simulink model "gm_wlanhdlTimeAndFrequencySynchronization"  (R2025a)
settings: Solver=FixedStepDiscrete  StartTime=0.0  StopTime=stopTime  RelTol=1e-3
InitFcn:
  | wlanFrontEndInit;
undefined symbols (not defined in the file or in its folder): a, b, c, Hd, wlanConfig
libraries: simulink x95, hdlsllib x16, hdlmdlgenlib x12, dspsrcs4 x3, dspsigops x3, dsphdlsigops2 x2, dsphdlfiltering2 x2
(part 10 of 11)

== system gm_wlanhdlTimeAndFrequencySynchronization/WLANTimeAndFrequencySynchronization/Fine CFO Estimation and Correction/Fine CFO Estimation/Iteration8 ==
  xin : Inport  OutDataTypeStr=fixdt(1, 32, 19)  SampleTime=6.25e-09
  yin : Inport  Port=2  OutDataTypeStr=fixdt(1, 32, 19)  SampleTime=6.25e-09
  zin : Inport  Port=3  OutDataTypeStr=fixdt(1, 34, 33)  SampleTime=6.25e-09
  lut_value : Inport  Port=4  OutDataTypeStr=fixdt(0, 31, 33)  SampleTime=6.25e-09
  idx : Inport  Port=5  OutDataTypeStr=fixdt(0, 6, 0)  SampleTime=6.25e-09
  MuxX : Switch  Criteria=u2 ~= 0  Threshold="fi(0,0,1,0,\"hex\",\"0\")"  OutDataTypeStr=fixdt(1, 32, 19)  SampleTime=6.25e-09  SaturateOnIntegerOverflow=off  InputSameDT=off
  MuxY : Switch  Criteria=u2 ~= 0  Threshold="fi(0,0,1,0,\"hex\",\"0\")"  OutDataTypeStr=fixdt(1, 32, 19)  SampleTime=6.25e-09  SaturateOnIntegerOverflow=off  InputSameDT=off
  MuxZ : Switch  Criteria=u2 ~= 0  Threshold="fi(0,0,1,0,\"hex\",\"0\")"  OutDataTypeStr=fixdt(1, 34, 33)  SampleTime=6.25e-09  SaturateOnIntegerOverflow=off  InputSameDT=off
  XAdder : Sum  OutDataTypeStr=fixdt(1, 32, 19)  SampleTime=6.25e-09
  XSubtractor : Sum  Inputs=+-  OutDataTypeStr=fixdt(1, 32, 19)  AccumDataTypeStr=fixdt(1, 32, 19)  SampleTime=6.25e-09
  YAdder : Sum  OutDataTypeStr=fixdt(1, 32, 19)  SampleTime=6.25e-09
  YSub : Sum  Inputs=+-  OutDataTypeStr=fixdt(1, 32, 19)  AccumDataTypeStr=fixdt(1, 32, 19)  SampleTime=6.25e-09
  ZAdder : Sum  OutDataTypeStr=fixdt(1, 34, 33)  SampleTime=6.25e-09
  ZSub : Sum  Inputs=+-  OutDataTypeStr=fixdt(1, 34, 33)  AccumDataTypeStr=fixdt(1, 34, 33)  SampleTime=6.25e-09
  compare : simulink/Logic and Bit Operations/Compare To Constant  relop=<  const=double(0)  OutDataTypeStr=boolean
  dynamic_shift : ArithShift  BitShiftNumberSource=Input port  BitShiftDirection=Right
      settings: InputPortMap=u0,p1
  dynamic_shift1 : ArithShift  BitShiftNumberSource=Input port  BitShiftDirection=Right
      settings: InputPortMap=u0,p1
  rd_{0..9} (10 alike) : Delay  DelayLength=double(1)  InitialCondition=0  SampleTime=6.25e-09
  xout : Outport  OutDataTypeStr=fixdt(1, 32, 19)  SampleTime=6.25e-09
  yout : Outport  Port=2  OutDataTypeStr=fixdt(1, 32, 19)  SampleTime=6.25e-09
  zout : Outport  Port=3  OutDataTypeStr=fixdt(1, 34, 33)  SampleTime=6.25e-09
  wires:
  rd_3/1 -> MuxZ/2, MuxY/2, MuxX/2
  rd_2/1 -> MuxX/1
  rd_6/1 -> MuxY/3
  ZAdder/1 -> rd_9/1
  ZSub/1 -> rd_8/1
  yin/1 -> rd_1/1
  MuxZ/1 -> zout/1
  MuxX/1 -> xout/1
  XAdder/1 -> rd_4/1
  idx/1 -> dynamic_shift/2, dynamic_shift1/2
  xin/1 -> rd_0/1
  rd_9/1 -> MuxZ/3
  zin/1 -> rd_7/1
  rd_1/1 -> compare/1, dynamic_shift1/1, YSub/1, YAdder/1
  rd_4/1 -> MuxX/3
  YSub/1 -> rd_6/1
  rd_0/1 -> dynamic_shift/1, XSubtractor/1, XAdder/1
  dynamic_shift/1 -> YAdder/2, YSub/2
  XSubtractor/1 -> rd_2/1
  compare/1 -> rd_3/1
  rd_8/1 -> MuxZ/1
  YAdder/1 -> rd_5/1
  rd_7/1 -> ZSub/1, ZAdder/1
  MuxY/1 -> yout/1
  rd_5/1 -> MuxY/1
  dynamic_shift1/1 -> XSubtractor/2, XAdder/2
  lut_value/1 -> ZSub/2, ZAdder/2

== system gm_wlanhdlTimeAndFrequencySynchronization/WLANTimeAndFrequencySynchronization/Fine CFO Estimation and Correction/Fine CFO Estimation/Iteration9 ==
  xin : Inport  OutDataTypeStr=fixdt(1, 32, 19)  SampleTime=6.25e-09
  yin : Inport  Port=2  OutDataTypeStr=fixdt(1, 32, 19)  SampleTime=6.25e-09
  zin : Inport  Port=3  OutDataTypeStr=fixdt(1, 34, 33)  SampleTime=6.25e-09
  lut_value : Inport  Port=4  OutDataTypeStr=fixdt(0, 31, 33)  SampleTime=6.25e-09
  idx : Inport  Port=5  OutDataTypeStr=fixdt(0, 6, 0)  SampleTime=6.25e-09
  MuxX : Switch  Criteria=u2 ~= 0  Threshold="fi(0,0,1,0,\"hex\",\"0\")"  OutDataTypeStr=fixdt(1, 32, 19)  SampleTime=6.25e-09  SaturateOnIntegerOverflow=off  InputSameDT=off
  MuxY : Switch  Criteria=u2 ~= 0  Threshold="fi(0,0,1,0,\"hex\",\"0\")"  OutDataTypeStr=fixdt(1, 32, 19)  SampleTime=6.25e-09  SaturateOnIntegerOverflow=off  InputSameDT=off
  MuxZ : Switch  Criteria=u2 ~= 0  Threshold="fi(0,0,1,0,\"hex\",\"0\")"  OutDataTypeStr=fixdt(1, 34, 33)  SampleTime=6.25e-09  SaturateOnIntegerOverflow=off  InputSameDT=off
  XAdder : Sum  OutDataTypeStr=fixdt(1, 32, 19)  SampleTime=6.25e-09
  XSubtractor : Sum  Inputs=+-  OutDataTypeStr=fixdt(1, 32, 19)  AccumDataTypeStr=fixdt(1, 32, 19)  SampleTime=6.25e-09
  YAdder : Sum  OutDataTypeStr=fixdt(1, 32, 19)  SampleTime=6.25e-09
  YSub : Sum  Inputs=+-  OutDataTypeStr=fixdt(1, 32, 19)  AccumDataTypeStr=fixdt(1, 32, 19)  SampleTime=6.25e-09
  ZAdder : Sum  OutDataTypeStr=fixdt(1, 34, 33)  SampleTime=6.25e-09
  ZSub : Sum  Inputs=+-  OutDataTypeStr=fixdt(1, 34, 33)  AccumDataTypeStr=fixdt(1, 34, 33)  SampleTime=6.25e-09
  compare : simulink/Logic and Bit Operations/Compare To Constant  relop=<  const=double(0)  OutDataTypeStr=boolean
  dynamic_shift : ArithShift  BitShiftNumberSource=Input port  BitShiftDirection=Right
      settings: InputPortMap=u0,p1
  dynamic_shift1 : ArithShift  BitShiftNumberSource=Input port  BitShiftDirection=Right
      settings: InputPortMap=u0,p1
  rd_{0..9} (10 alike) : Delay  DelayLength=double(1)  InitialCondition=0  SampleTime=6.25e-09
  xout : Outport  OutDataTypeStr=fixdt(1, 32, 19)  SampleTime=6.25e-09
  yout : Outport  Port=2  OutDataTypeStr=fixdt(1, 32, 19)  SampleTime=6.25e-09
  zout : Outport  Port=3  OutDataTypeStr=fixdt(1, 34, 33)  SampleTime=6.25e-09
  wires:
  MuxX/1 -> xout/1
  MuxZ/1 -> zout/1
  rd_4/1 -> MuxX/3
  rd_3/1 -> MuxZ/2, MuxX/2, MuxY/2
  rd_5/1 -> MuxY/1
  rd_8/1 -> MuxZ/1
  MuxY/1 -> yout/1
  XAdder/1 -> rd_4/1
  rd_9/1 -> MuxZ/3
  XSubtractor/1 -> rd_2/1
  yin/1 -> rd_1/1
  zin/1 -> rd_7/1
  YAdder/1 -> rd_5/1
  rd_1/1 -> compare/1, dynamic_shift1/1, YAdder/1, YSub/1
  rd_6/1 -> MuxY/3
  idx/1 -> dynamic_shift1/2, dynamic_shift/2
  rd_2/1 -> MuxX/1
  rd_7/1 -> ZSub/1, ZAdder/1
  lut_value/1 -> ZAdder/2, ZSub/2
  dynamic_shift1/1 -> XAdder/2, XSubtractor/2
  YSub/1 -> rd_6/1
  xin/1 -> rd_0/1
  rd_0/1 -> dynamic_shift/1, XSubtractor/1, XAdder/1
  compare/1 -> rd_3/1
  dynamic_shift/1 -> YSub/2, YAdder/2
  ZSub/1 -> rd_8/1
  ZAdder/1 -> rd_9/1

== system gm_wlanhdlTimeAndFrequencySynchronization/WLANTimeAndFrequencySynchronization/Fine CFO Estimation and Correction/Fine CFO Estimation/QuadrantCorrection ==
  zin : Inport  OutDataTypeStr=fixdt(1, 34, 33)  SampleTime=6.25e-09
  QA_Control : Inport  Port=2  OutDataTypeStr=fixdt(0, 5, 0)  SampleTime=6.25e-09
  Negation : Gain  Gain="fi(0,1,2,0,\"hex\",\"3\")"  ParamDataTypeStr=fixdt(1, 2, 0)  OutDataTypeStr=fixdt(1, 34, 33)  SampleTime=6.25e-09
  adder : Sum  OutDataTypeStr=fixdt(1, 34, 33)  SampleTime=6.25e-09
  dtc : hdlmdlgenlib/Buffer
  extract : simulink/Logic and Bit Operations/Extract Bits  bitsToExtract=Range of bits  numBits=8  bitIdxRange=[2 2]  outScalingMode=Treat bit field as an integer
  extract1 : simulink/Logic and Bit Operations/Extract Bits  bitsToExtract=Range of bits  numBits=8  bitIdxRange=[0 1]  outScalingMode=Treat bit field as an integer
  mux : MultiPortSwitch  DataPortOrder=Zero-based contiguous  Inputs=2  DiagnosticForDefault=None  zeroidx=on  OutDataTypeStr=fixdt(1, 34, 33)  SampleTime=6.25e-09  SaturateOnIntegerOverflow=off  InputSameDT=off
  mux1 : MultiPortSwitch  DataPortOrder=Zero-based contiguous  Inputs=4  DiagnosticForDefault=None  zeroidx=on  OutDataTypeStr=fixdt(1, 34, 33)  SampleTime=6.25e-09  SaturateOnIntegerOverflow=off  InputSameDT=off
  mux2 : MultiPortSwitch  DataPortOrder=Zero-based contiguous  Inputs=2  DiagnosticForDefault=None  zeroidx=on  OutDataTypeStr=fixdt(1, 34, 33)  SampleTime=6.25e-09  SaturateOnIntegerOverflow=off  InputSameDT=off
  mux3 : MultiPortSwitch  DataPortOrder=Zero-based contiguous  Inputs=2  DiagnosticForDefault=None  zeroidx=on  OutDataTypeStr=fixdt(1, 34, 33)  SampleTime=6.25e-09  SaturateOnIntegerOverflow=off  InputSameDT=off
  mux6out_wire : hdlmdlgenlib/Buffer
  pidivtwoconstant : Constant  Value=0.5  OutDataTypeStr=fixdt(1, 34, 33)  SampleTime=6.25e-09
  pidivtwoconstant1 : Constant  Value=0.999999999883584678173065185546875  OutDataTypeStr=fixdt(1, 34, 33)  SampleTime=6.25e-09
  pidivtwoconstant2 : Constant  Value=-1  OutDataTypeStr=fixdt(1, 34, 33)  SampleTime=6.25e-09
  pidivtwoconstant3 : Constant  Value=0  OutDataTypeStr=fixdt(1, 34, 33)  SampleTime=6.25e-09
  pidivtwosub : Sum  Inputs=+-  OutDataTypeStr=fixdt(1, 34, 33)  AccumDataTypeStr=fixdt(1, 34, 33)  SampleTime=6.25e-09
  rd_{0,2..3,6..7} (5 alike) : Delay  DelayLength=double(1)  InitialCondition=0  SampleTime=6.25e-09
  rd_{1,4..5,8..9} (5 alike) : Delay  DelayLength=double(2)  InitialCondition=0  SampleTime=6.25e-09
  slice : hdlsllib/Logic and Bit Operations/Bit Slice  lidx=double(3)  ridx=double(3)
  slice1 : hdlsllib/Logic and Bit Operations/Bit Slice  lidx=double(4)  ridx=double(4)
  subfmux : Sum  Inputs=+-  OutDataTypeStr=fixdt(1, 34, 33)  AccumDataTypeStr=fixdt(1, 34, 33)  SampleTime=6.25e-09
  zout : Outport  OutDataTypeStr=fixdt(1, 34, 33)  SampleTime=6.25e-09
  wires:
  mux6out_wire/1 -> zout/1
  pidivtwoconstant2/1 -> adder/1
  Negation/1 -> rd_7/1
  extract1/1 -> rd_5/1
  pidivtwosub/1 -> mux/2
  rd_2/1 -> dtc/1
  extract/1 -> mux/1
  slice1/1 -> rd_1/1
  rd_7/1 -> mux1/3
  mux/1 -> rd_3/1, adder/2, subfmux/2
  rd_5/1 -> mux1/1
  rd_9/1 -> mux1/5
  mux1/1 -> mux2/2
  dtc/1 -> pidivtwosub/2, mux/3
  slice/1 -> rd_4/1
  pidivtwoconstant/1 -> pidivtwosub/1
  mux3/1 -> mux6out_wire/1
  rd_0/1 -> extract/1, slice/1, slice1/1, extract1/1
  rd_6/1 -> mux1/2
  QA_Control/1 -> rd_0/1
  rd_3/1 -> rd_6/1, Negation/1
  pidivtwoconstant1/1 -> subfmux/1, mux2/3
  adder/1 -> rd_9/1
  pidivtwoconstant3/1 -> mux3/3
  subfmux/1 -> rd_8/1
  rd_8/1 -> mux1/4
  zin/1 -> rd_2/1
  rd_1/1 -> mux3/1
  rd_4/1 -> mux2/1
  mux2/1 -> mux3/2

== system gm_wlanhdlTimeAndFrequencySynchronization/WLANTimeAndFrequencySynchronization/Fine CFO Estimation and Correction/Fine CFO Estimation/QuadrantMapper ==
  xin : Inport  OutDataTypeStr=fixdt(1, 32, 19)  SampleTime=5e-08
  yin : Inport  Port=2  OutDataTypeStr=fixdt(1, 32, 19)  SampleTime=5e-08
  Delayin1 : UnitDelay  InitialCondition=double(0)  SampleTime=5e-08
  Delayin11 : RateTransition  InitialCondition=double(0)  OutPortSampleTimeOpt=Multiple of input port sample time  OutPortSampleTimeMultiple=8
  Delayin2 : UnitDelay  InitialCondition=double(0)  SampleTime=5e-08
  Delayin21 : RateTransition  InitialCondition=double(0)  OutPortSampleTimeOpt=Multiple of input port sample time  OutPortSampleTimeMultiple=8
  DelayxAbs : RateTransition  InitialCondition=double(0)  OutPortSampleTimeOpt=Multiple of input port sample time  OutPortSampleTimeMultiple=8
  DelayxAbs_absorbed : Delay  DelayLength=0
  DelayyAbs : RateTransition  InitialCondition=double(0)  OutPortSampleTimeOpt=Multiple of input port sample time  OutPortSampleTimeMultiple=8
  DelayyAbs_absorbed : Delay  DelayLength=0
  abs : Abs  SampleTime=6.25e-09  OutDataTypeStr=fixdt(1, 32, 19)  SaturateOnIntegerOverflow=off
  abs1 : Abs  SampleTime=6.25e-09  OutDataTypeStr=fixdt(1, 32, 19)  SaturateOnIntegerOverflow=off
  and : Logic  AllPortsSameDT=off  OutDataTypeStr=fixdt(0, 1, 0)  SampleTime=6.25e-09
  and1 : Logic  AllPortsSameDT=off  OutDataTypeStr=fixdt(0, 1, 0)  SampleTime=6.25e-09
  compare : simulink/Logic and Bit Operations/Compare To Constant  relop=<  const=double(0)  OutDataTypeStr=boolean
  compare1 : simulink/Logic and Bit Operations/Compare To Constant  relop===  const=double(0)  OutDataTypeStr=boolean
  compare2 : simulink/Logic and Bit Operations/Compare To Constant  relop=>=  const=double(0)  OutDataTypeStr=boolean
  compare3 : simulink/Logic and Bit Operations/Compare To Constant  relop=<  const=double(0)  OutDataTypeStr=boolean
  concatQCControl : hdlsllib/Logic and Bit Operations/Bit Concat  numInputs=5
  crp_out_delay : Delay  DelayLength=double(1)  InitialCondition=0  SampleTime=6.25e-09
  crp_out_delay1 : Delay  DelayLength=double(1)  InitialCondition=0  SampleTime=6.25e-09
  dtc : hdlmdlgenlib/Buffer
  dtc1 : hdlmdlgenlib/Buffer
  in0_repeat : RateTransition  Integrity=off  Deterministic=off  OutPortSampleTimeOpt=Multiple of input port sample time  OutPortSampleTimeMultiple=1/8
  in0_repeat1 : RateTransition  Integrity=off  Deterministic=off  OutPortSampleTimeOpt=Multiple of input port sample time  OutPortSampleTimeMultiple=1/8
  in1_repeat : RateTransition  Integrity=off  Deterministic=off  OutPortSampleTimeOpt=Multiple of input port sample time  OutPortSampleTimeMultiple=1/8
  in1_repeat1 : RateTransition  Integrity=off  Deterministic=off  OutPortSampleTimeOpt=Multiple of input port sample time  OutPortSampleTimeMultiple=1/8
  in2_repeat : RateTransition  Integrity=off  Deterministic=off  OutPortSampleTimeOpt=Multiple of input port sample time  OutPortSampleTimeMultiple=1/8
  in3_repeat : RateTransition  Integrity=off  Deterministic=off  OutPortSampleTimeOpt=Multiple of input port sample time  OutPortSampleTimeMultiple=1/8
  mux : MultiPortSwitch  DataPortOrder=Zero-based contiguous  Inputs=2  DiagnosticForDefault=None  zeroidx=on  OutDataTypeStr=fixdt(1, 32, 19)  SampleTime=6.25e-09  SaturateOnIntegerOverflow=off  InputSameDT=off
  mux1 : MultiPortSwitch  DataPortOrder=Zero-based contiguous  Inputs=2  DiagnosticForDefault=None  zeroidx=on  OutDataTypeStr=fixdt(1, 32, 19)  SampleTime=6.25e-09  SaturateOnIntegerOverflow=off  InputSameDT=off
  qcControl_wire : hdlmdlgenlib/Buffer
  rd_{0..10,41} (12 alike) : Delay  DelayLength=double(1)  InitialCondition=0  SampleTime=6.25e-09
  rd_01 : Delay  DelayLength=double(1)  InitialCondition=0  SampleTime=6.25e-09
  relop : RelationalOperator  Operator=>  OutDataTypeStr=fixdt(0, 1, 0)  SampleTime=6.25e-09
  xout : Outport  OutDataTypeStr=fixdt(1, 32, 19)  SampleTime=6.25e-09
  yout : Outport  Port=2  OutDataTypeStr=fixdt(1, 32, 19)  SampleTime=6.25e-09
  QA_Control : Outport  Port=3  OutDataTypeStr=fixdt(0, 5, 0)  SampleTime=6.25e-09
  wires:
  rd_9/1 -> mux/2, mux1/3
  rd_7/1 -> concatQCControl/3, mux/1, mux1/1
  and/1 -> concatQCControl/2
  mux/1 -> dtc/1
  and1/1 -> concatQCControl/1
  relop/1 -> rd_7/1
  rd_10/1 -> mux/3, mux1/2
  rd_6/1 -> relop/2, rd_10/1
  rd_4/1 -> and/2, concatQCControl/4
  crp_out_delay/1 -> DelayyAbs/1
  abs/1 -> crp_out_delay/1
  concatQCControl/1 -> qcControl_wire/1
  abs1/1 -> crp_out_delay1/1
  yin/1 -> in0_repeat1/1
  rd_3/1 -> and1/2
  DelayxAbs/1 -> DelayxAbs_absorbed/1
  Delayin11/1 -> Delayin1/1
  rd_41/1 -> abs1/1
  compare1/1 -> rd_1/1
  DelayyAbs/1 -> DelayyAbs_absorbed/1
  dtc/1 -> yout/1
  crp_out_delay1/1 -> DelayxAbs/1
  in0_repeat1/1 -> Delayin21/1, rd_01/1
  in1_repeat1/1 -> rd_41/1, Delayin11/1
  rd_01/1 -> abs/1
  dtc1/1 -> xout/1
  rd_8/1 -> concatQCControl/5
  rd_1/1 -> and/1, and1/1
  Delayin2/1 -> in1_repeat/1
  xin/1 -> in1_repeat1/1
  in3_repeat/1 -> rd_6/1
  Delayin1/1 -> in0_repeat/1
  in0_repeat/1 -> rd_2/1
  qcControl_wire/1 -> QA_Control/1
  in1_repeat/1 -> rd_0/1
  compare2/1 -> rd_3/1
  DelayxAbs_absorbed/1 -> in2_repeat/1
  DelayyAbs_absorbed/1 -> in3_repeat/1
  rd_2/1 -> compare/1, compare2/1
  rd_0/1 -> compare1/1, compare3/1
  in2_repeat/1 -> rd_5/1
  compare/1 -> rd_4/1
  mux1/1 -> dtc1/1
  compare3/1 -> rd_8/1
  Delayin21/1 -> Delayin2/1
  rd_5/1 -> relop/1, rd_9/1

== system gm_wlanhdlTimeAndFrequencySynchronization/WLANTimeAndFrequencySynchronization/Fine CFO Estimation and Correction/Fine CFO Estimation/sample FreqOff ==
  freqOffIn : Inport  OutDataTypeStr=fixdt(1, 34, 33)  PortDimensions=1  SampleTime=5e-08
  enb : Inport  Port=2  OutDataTypeStr=boolean  PortDimensions=1  SampleTime=5e-08
  rst : Inport  Port=3  OutDataTypeStr=boolean  PortDimensions=1  SampleTime=5e-08
  Sample FreqOff : MATLAB Function  TreatAsAtomicUnit=on
  freqOffOut : Outport  SampleTime=5e-08  VectorParamsAs1DForOutWhenUnconnected=off
  wires:
  freqOffIn/1 -> Sample FreqOff/1(freqOffIn)
  enb/1 -> Sample FreqOff/2(enb)
  rst/1 -> Sample FreqOff/3(rst)
  Sample FreqOff/1(freqOffOut) -> freqOffOut/1

== system gm_wlanhdlTimeAndFrequencySynchronization/WLANTimeAndFrequencySynchronization/Fine Time Sync/Correlator/MagnitudeSquared ==
  dataIn : Inport  OutDataTypeStr=fixdt(1, 37, 26)  PortDimensions=1  SampleTime=5e-08
      settings: SignalType=complex
  validIn : Inport  Port=2  OutDataTypeStr=boolean  PortDimensions=1  SampleTime=5e-08
  Add : Sum  OutDataTypeStr=fixdt(1, 33, 16)  AccumDataTypeStr=fixdt(1, 33, 16)  SampleTime=6.25e-09
  Complex to Real-Imag : ComplexToRealImag  SampleTime=5e-08
  Data Type  Conversion : DataTypeConversion  OutDataTypeStr=fixdt(1, 16, 8)  SampleTime=5e-08  SaturateOnIntegerOverflow=off  RndMeth=Floor
  Data Type  Conversion1 : DataTypeConversion  OutDataTypeStr=fixdt(1, 32, 15)  SampleTime=6.25e-09  SaturateOnIntegerOverflow=off  RndMeth=Floor
  Delay1 : Delay  DelayLength=double(2)  InitialCondition=0  SampleTime=5e-08
  Delay3 : Delay  DelayLength=double(2)  InitialCondition=0  SampleTime=5e-08
  Delay4 : RateTransition  InitialCondition=double(0)  OutPortSampleTimeOpt=Multiple of input port sample time  OutPortSampleTimeMultiple=8
  Delay4_absorbed : Delay  DelayLength=0
  Delay5 : RateTransition  InitialCondition=double(0)  OutPortSampleTimeOpt=Multiple of input port sample time  OutPortSampleTimeMultiple=8
  Delay5_absorbed : Delay  DelayLength=0
  Delay6 : Delay  DelayLength=double(3)  InitialCondition=0  SampleTime=5e-08
  Delay61 : RateTransition  InitialCondition=double(0)  OutPortSampleTimeOpt=Multiple of input port sample time  OutPortSampleTimeMultiple=8
  HwModeRegister{,1..3} (4 alike) : Delay  DelayLength=double(1)  InitialCondition=0  SampleTime=6.25e-09
  PipelineRegister : Delay  DelayLength=double(1)  InitialCondition=0  SampleTime=6.25e-09
  PipelineRegister1 : Delay  DelayLength=double(1)  InitialCondition=0  SampleTime=6.25e-09
  Product1 : Product  Inputs=**  OutDataTypeStr=fixdt(1, 32, 16)  SampleTime=6.25e-09
  Product4 : Product  Inputs=**  OutDataTypeStr=fixdt(1, 32, 16)  SampleTime=6.25e-09
  crp_out_delay : Delay  DelayLength=double(1)  InitialCondition=0  SampleTime=6.25e-09
  crp_out_delay1 : Delay  DelayLength=double(1)  InitialCondition=0  SampleTime=6.25e-09
  in0_repeat : RateTransition  Integrity=off  Deterministic=off  OutPortSampleTimeOpt=Multiple of input port sample time  OutPortSampleTimeMultiple=1/8
  in0_repeat1 : RateTransition  Integrity=off  Deterministic=off  OutPortSampleTimeOpt=Multiple of input port sample time  OutPortSampleTimeMultiple=1/8
  in1_repeat : RateTransition  Integrity=off  Deterministic=off  OutPortSampleTimeOpt=Multiple of input port sample time  OutPortSampleTimeMultiple=1/8
  in1_repeat1 : RateTransition  Integrity=off  Deterministic=off  OutPortSampleTimeOpt=Multiple of input port sample time  OutPortSampleTimeMultiple=1/8
  in2_repeat : RateTransition  Integrity=off  Deterministic=off  OutPortSampleTimeOpt=Multiple of input port sample time  OutPortSampleTimeMultiple=1/8
  in2_repeat1 : RateTransition  Integrity=off  Deterministic=off  OutPortSampleTimeOpt=Multiple of input port sample time  OutPortSampleTimeMultiple=1/8
  in3_repeat : RateTransition  Integrity=off  Deterministic=off  OutPortSampleTimeOpt=Multiple of input port sample time  OutPortSampleTimeMultiple=1/8
  rd_{0..4,11} (6 alike) : Delay  DelayLength=double(1)  InitialCondition=0  SampleTime=6.25e-09
  dataOut : Outport  SampleTime=6.25e-09  VectorParamsAs1DForOutWhenUnconnected=off
  validOut : Outport  Port=2  SampleTime=5e-08  VectorParamsAs1DForOutWhenUnconnected=off
  wires:
  in2_repeat/1 -> rd_2/1
  in1_repeat/1 -> rd_1/1
  Delay5_absorbed/1 -> in2_repeat/1
  in2_repeat1/1 -> rd_3/1
  rd_11/1 -> HwModeRegister1/1
  Delay6/1 -> validOut/1
  Data Type  Conversion1/1 -> dataOut/1
  Delay3/1 -> in2_repeat1/1, in3_repeat/1
  in0_repeat/1 -> Delay61/1
  HwModeRegister1/1 -> Product4/2
  in0_repeat1/1 -> rd_0/1
  crp_out_delay/1 -> Delay4/1
  Delay4_absorbed/1 -> in1_repeat/1
  Delay5/1 -> Delay5_absorbed/1
  in3_repeat/1 -> rd_4/1
  Delay1/1 -> in0_repeat1/1, in1_repeat1/1
  Complex to Real-Imag/2 -> Delay3/1
  Complex to Real-Imag/1 -> Delay1/1
  Add/1 -> Data Type  Conversion1/1
  dataIn/1 -> Data Type  Conversion/1
  Data Type  Conversion/1 -> Complex to Real-Imag/1
  rd_2/1 -> Add/2
  validIn/1 -> in0_repeat/1
  HwModeRegister3/1 -> Product1/2
  HwModeRegister/1 -> Product4/1
  crp_out_delay1/1 -> Delay5/1
  in1_repeat1/1 -> rd_11/1
  Delay61/1 -> Delay6/1
  Product1/1 -> PipelineRegister1/1
  PipelineRegister1/1 -> crp_out_delay1/1
  rd_0/1 -> HwModeRegister/1
  rd_1/1 -> Add/1
  rd_3/1 -> HwModeRegister2/1
  rd_4/1 -> HwModeRegister3/1
  Delay4/1 -> Delay4_absorbed/1
  HwModeRegister2/1 -> Product1/1
  PipelineRegister/1 -> crp_out_delay/1
  Product4/1 -> PipelineRegister/1

== system gm_wlanhdlTimeAndFrequencySynchronization/WLANTimeAndFrequencySynchronization/Fine Time Sync/Correlator/corrFilter ==
  dataIn : Inport  OutDataTypeStr=fixdt(1, 16, 12)  PortDimensions=1  SampleTime=5e-08
      settings: SignalType=complex
  validIn : Inport  Port=2  OutDataTypeStr=boolean  PortDimensions=1  SampleTime=5e-08
  rst : Inport  Port=3  OutDataTypeStr=boolean  PortDimensions=1  SampleTime=5e-08
  C1 : dsphdlfiltering2/Discrete FIR Filter  NumeratorSource=Property  Numerator=conj(flipud(wlanConfig.lltf(1:wlanConfig.corrLen))).'  NumeratorPrototype=[ 0.5, 0.5 ]  FilterStructure=Partly serial systolic  SerializationOption=Minimum number of cycles between valid input samples  NumCycles=filterUpsampleFactor  NumberOfMultipliers=2  SimulateUsing=Code generation  roundingMode=Floor  overflowMode=off  CoefficientsDataTypeStr=fixdt(1,16,14)  ResetInputPort=on  HDLGlobalReset=off  CoeffMultiplier=Multiplier  UseMultForPow2Coeff=on  FrameInputSymmOptim=off
  C1_term2 : Terminator
  Delay : Delay  DelayLength=double(7)  InitialCondition=0  SampleTime=6.25e-09
  Delay1 : Delay  DelayLength=double(7)  InitialCondition=0  SampleTime=6.25e-09
  Downsample : DownSample  N=double(8)  phase=double(0)  RateOptions=Allow multirate processing  AllowArbitraryFixedInput=on
  Downsample1 : DownSample  N=double(8)  phase=double(0)  RateOptions=Allow multirate processing  AllowArbitraryFixedInput=on
  PipelineRegister : Delay  DelayLength=double(1)  InitialCondition=0  SampleTime=5e-08
  PipelineRegister1 : Delay  DelayLength=double(1)  InitialCondition=0  SampleTime=5e-08
  Upsample : dspsigops/Upsample  FactorSource=Dialog parameter  N=double(8)  Nmax=16  phase=double(0)  RateOptions=Allow multirate processing  ic=0  mode=Unused parameter value
  Upsample1 : dspsigops/Upsample  FactorSource=Dialog parameter  N=double(8)  Nmax=16  phase=double(0)  RateOptions=Allow multirate processing  ic=0  mode=Unused parameter value
  Upsample2 : dspsigops/Upsample  FactorSource=Dialog parameter  N=double(8)  Nmax=16  phase=double(0)  RateOptions=Allow multirate processing  ic=0  mode=Unused parameter value
  dataOut : Outport  SampleTime=5e-08
  validOut : Outport  Port=2  SampleTime=5e-08
  wires:
  PipelineRegister/1 -> validOut/1
  PipelineRegister1/1 -> dataOut/1
  dataIn/1 -> Upsample/1
  rst/1 -> Upsample2/1
  C1/1 -> Delay/1
  Upsample/1 -> C1/1
  Upsample2/1 -> C1/3
  C1/2 -> Delay1/1
  Delay/1 -> Downsample/1
  validIn/1 -> Upsample1/1
  Delay1/1 -> Downsample1/1
  Upsample1/1 -> C1/2
  Downsample/1 -> PipelineRegister1/1
  C1/3 -> C1_term2/1
  Downsample1/1 -> PipelineRegister/1

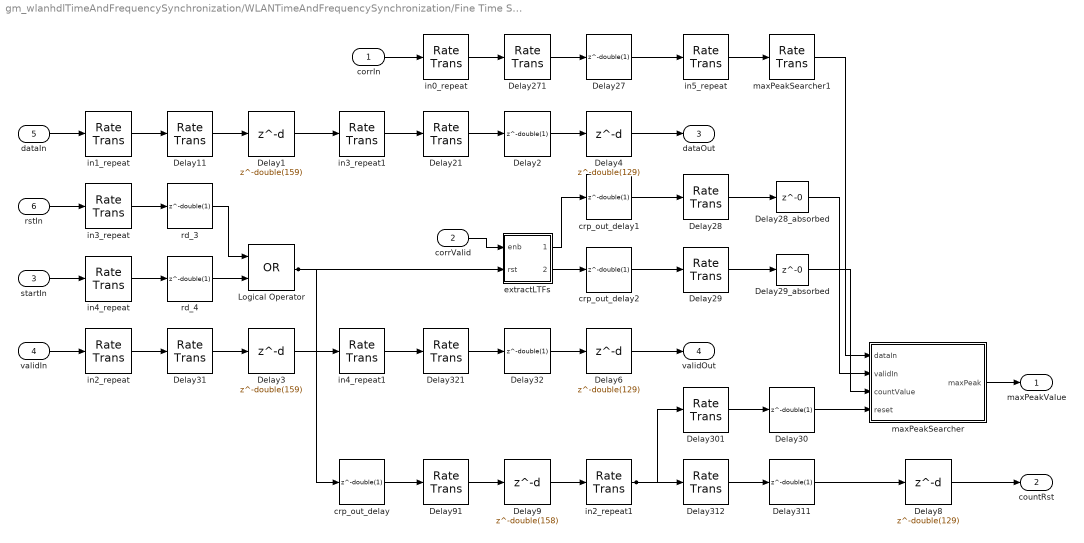
== system gm_wlanhdlTimeAndFrequencySynchronization/WLANTimeAndFrequencySynchronization/Fine Time Sync/Peak Searcher/maxPeakSearcher ==
  corrIn : Inport  OutDataTypeStr=fixdt(1, 32, 15)  PortDimensions=1  SampleTime=5e-08
  corrValid : Inport  Port=2  OutDataTypeStr=boolean  PortDimensions=1  SampleTime=5e-08
  startIn : Inport  Port=3  OutDataTypeStr=boolean  PortDimensions=1  SampleTime=5e-08
  validIn : Inport  Port=4  OutDataTypeStr=boolean  PortDimensions=1  SampleTime=5e-08
  dataIn : Inport  Port=5  OutDataTypeStr=fixdt(1, 16, 12)  PortDimensions=1  SampleTime=5e-08
      settings: SignalType=complex
  rstIn : Inport  Port=6  OutDataTypeStr=boolean  PortDimensions=1  SampleTime=5e-08
  Delay1 : Delay  DelayLength=double(159)  InitialCondition=0  SampleTime=5e-08
  Delay{11,21,28..29,31,91,271,301,312,321} (10 alike) : RateTransition  InitialCondition=double(0)  OutPortSampleTimeOpt=Multiple of input port sample time  OutPortSampleTimeMultiple=8
  Delay{2,27,30,32,311} (5 alike) : Delay  DelayLength=double(1)  InitialCondition=0  SampleTime=5e-08
  Delay28_absorbed : Delay  DelayLength=0
  Delay29_absorbed : Delay  DelayLength=0
  Delay3 : Delay  DelayLength=double(159)  InitialCondition=0  SampleTime=5e-08
  Delay4 : Delay  DelayLength=double(129)  InitialCondition=0  SampleTime=5e-08
  Delay6 : Delay  DelayLength=double(129)  InitialCondition=0  SampleTime=5e-08
  Delay8 : Delay  DelayLength=double(129)  InitialCondition=0  SampleTime=5e-08
  Delay9 : Delay  DelayLength=double(158)  InitialCondition=0  SampleTime=5e-08
  Logical Operator : Logic  Operator=OR  AllPortsSameDT=off  OutDataTypeStr=boolean  SampleTime=6.25e-09
  crp_out_delay : Delay  DelayLength=double(1)  InitialCondition=0  SampleTime=6.25e-09
  crp_out_delay1 : Delay  DelayLength=double(1)  InitialCondition=0  SampleTime=6.25e-09
  crp_out_delay2 : Delay  DelayLength=double(1)  InitialCondition=0  SampleTime=6.25e-09
  extractLTFs : Subsystem
  in0_repeat : RateTransition  Integrity=off  Deterministic=off  OutPortSampleTimeOpt=Multiple of input port sample time  OutPortSampleTimeMultiple=1/8
  in1_repeat : RateTransition  Integrity=off  Deterministic=off  OutPortSampleTimeOpt=Multiple of input port sample time  OutPortSampleTimeMultiple=1/8
  in2_repeat : RateTransition  Integrity=off  Deterministic=off  OutPortSampleTimeOpt=Multiple of input port sample time  OutPortSampleTimeMultiple=1/8
  in2_repeat1 : RateTransition  Integrity=off  Deterministic=off  OutPortSampleTimeOpt=Multiple of input port sample time  OutPortSampleTimeMultiple=1/8
  in3_repeat : RateTransition  Integrity=off  Deterministic=off  OutPortSampleTimeOpt=Multiple of input port sample time  OutPortSampleTimeMultiple=1/8
  in3_repeat1 : RateTransition  Integrity=off  Deterministic=off  OutPortSampleTimeOpt=Multiple of input port sample time  OutPortSampleTimeMultiple=1/8
  in4_repeat : RateTransition  Integrity=off  Deterministic=off  OutPortSampleTimeOpt=Multiple of input port sample time  OutPortSampleTimeMultiple=1/8
  in4_repeat1 : RateTransition  Integrity=off  Deterministic=off  OutPortSampleTimeOpt=Multiple of input port sample time  OutPortSampleTimeMultiple=1/8
  in5_repeat : RateTransition  Integrity=off  Deterministic=off  OutPortSampleTimeOpt=Multiple of input port sample time  OutPortSampleTimeMultiple=1/8
  maxPeakSearcher : Subsystem
  maxPeakSearcher1 : RateTransition  InitialCondition=double(0)  OutPortSampleTimeOpt=Multiple of input port sample time  OutPortSampleTimeMultiple=8
  rd_3 : Delay  DelayLength=double(1)  InitialCondition=0  SampleTime=6.25e-09
  rd_4 : Delay  DelayLength=double(1)  InitialCondition=0  SampleTime=6.25e-09
  maxPeakValue : Outport  SampleTime=5e-08
  countRst : Outport  Port=2  SampleTime=5e-08
  dataOut : Outport  Port=3  SampleTime=5e-08
  validOut : Outport  Port=4  SampleTime=5e-08
  wires:
  Delay311/1 -> Delay8/1
  Delay28_absorbed/1 -> maxPeakSearcher/2(validIn)
  maxPeakSearcher1/1 -> maxPeakSearcher/1(dataIn)
  Delay312/1 -> Delay311/1
  Delay301/1 -> Delay30/1
  Delay28/1 -> Delay28_absorbed/1
  in2_repeat1/1 -> Delay312/1, Delay301/1
  Delay29_absorbed/1 -> maxPeakSearcher/3(countValue)
  Delay6/1 -> validOut/1
  Delay27/1 -> in5_repeat/1
  Delay9/1 -> in2_repeat1/1
  Delay8/1 -> countRst/1
  Delay31/1 -> Delay3/1
  maxPeakSearcher/1(maxPeak) -> maxPeakValue/1
  crp_out_delay1/1 -> Delay28/1
  rd_4/1 -> Logical Operator/2
  dataIn/1 -> in1_repeat/1
  Delay2/1 -> Delay4/1
  in2_repeat/1 -> Delay31/1
  Delay30/1 -> maxPeakSearcher/4(reset)
  Delay4/1 -> dataOut/1
  startIn/1 -> in4_repeat/1
  in3_repeat1/1 -> Delay21/1
  crp_out_delay2/1 -> Delay29/1
  in1_repeat/1 -> Delay11/1
  Delay29/1 -> Delay29_absorbed/1
  Delay32/1 -> Delay6/1
  Delay3/1 -> in4_repeat1/1
  in4_repeat/1 -> rd_4/1
  validIn/1 -> in2_repeat/1
  rstIn/1 -> in3_repeat/1
  Delay1/1 -> in3_repeat1/1
  extractLTFs/2(count) -> crp_out_delay2/1
  Logical Operator/1 -> crp_out_delay/1, extractLTFs/2(rst)
  corrIn/1 -> in0_repeat/1
  Delay271/1 -> Delay27/1
  in5_repeat/1 -> maxPeakSearcher1/1
  in4_repeat1/1 -> Delay321/1
  crp_out_delay/1 -> Delay91/1
  in0_repeat/1 -> Delay271/1
  Delay321/1 -> Delay32/1
  Delay11/1 -> Delay1/1
  Delay21/1 -> Delay2/1
  in3_repeat/1 -> rd_3/1
  rd_3/1 -> Logical Operator/1
  corrValid/1 -> extractLTFs/1(enb)
  Delay91/1 -> Delay9/1
  extractLTFs/1(valid) -> crp_out_delay1/1

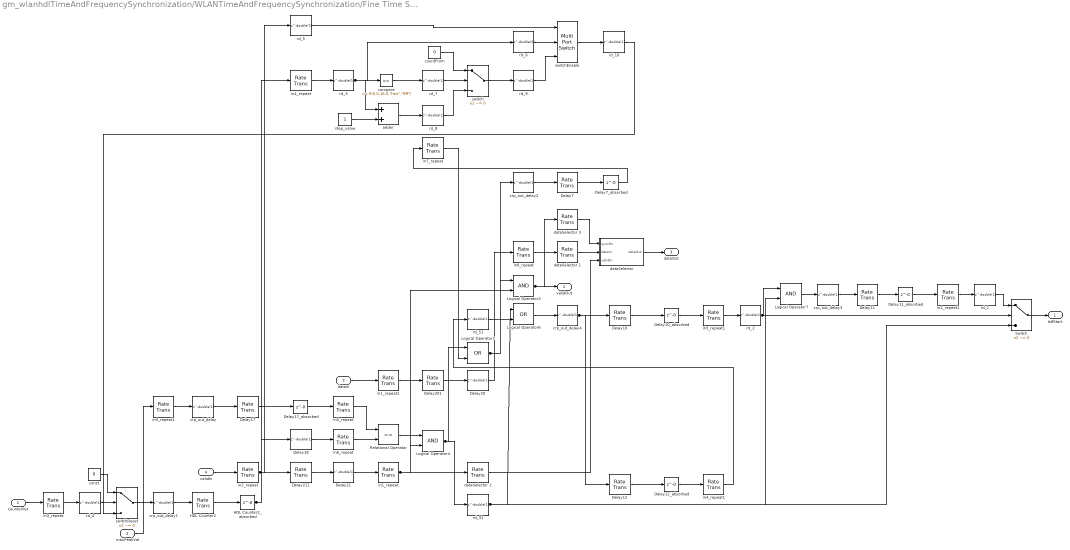
== system gm_wlanhdlTimeAndFrequencySynchronization/WLANTimeAndFrequencySynchronization/Fine Time Sync/Peak Searcher/peakDetector ==
  maxPeakVal : Inport  OutDataTypeStr=uint16  PortDimensions=1  SampleTime=5e-08
  counterRst : Inport  Port=2  OutDataTypeStr=boolean  PortDimensions=1  SampleTime=5e-08
  dataIn : Inport  Port=3  OutDataTypeStr=fixdt(1, 16, 12)  PortDimensions=1  SampleTime=5e-08
      settings: SignalType=complex
  validIn : Inport  Port=4  OutDataTypeStr=boolean  PortDimensions=1  SampleTime=5e-08
  Delay{7,10..12,17,201,211} (7 alike) : RateTransition  InitialCondition=double(0)  OutPortSampleTimeOpt=Multiple of input port sample time  OutPortSampleTimeMultiple=8
  Delay10_absorbed : Delay  DelayLength=0
  Delay11_absorbed : Delay  DelayLength=0
  Delay12_absorbed : Delay  DelayLength=0
  Delay17_absorbed : Delay  DelayLength=0
  Delay18 : Delay  DelayLength=double(1)  InitialCondition=0  SampleTime=5e-08
  Delay20 : Delay  DelayLength=double(1)  InitialCondition=0  SampleTime=5e-08
  Delay21 : Delay  DelayLength=double(1)  InitialCondition=0  SampleTime=5e-08
  Delay7_absorbed : Delay  DelayLength=0
  HDL Counter2 : RateTransition  InitialCondition=double(0)  OutPortSampleTimeOpt=Multiple of input port sample time  OutPortSampleTimeMultiple=8
  HDL Counter2_absorbed : Delay  DelayLength=0
  Logical Operator2 : Logic  Operator=OR  AllPortsSameDT=off  OutDataTypeStr=boolean  SampleTime=6.25e-09
  Logical Operator3 : Logic  AllPortsSameDT=off  OutDataTypeStr=boolean  SampleTime=6.25e-09
  Logical Operator4 : Logic  AllPortsSameDT=off  OutDataTypeStr=boolean  SampleTime=6.25e-09
  Logical Operator6 : Logic  Operator=OR  AllPortsSameDT=off  OutDataTypeStr=boolean  SampleTime=6.25e-09
  Logical Operator7 : Logic  AllPortsSameDT=off  OutDataTypeStr=boolean  SampleTime=6.25e-09
  Relational Operator : RelationalOperator  Operator===  OutDataTypeStr=boolean  SampleTime=6.25e-09  InputSameDT=off
  Switch : Switch  Criteria=u2 ~= 0  Threshold="fi(0,0,1,0,\"hex\",\"0\")"  OutDataTypeStr=boolean  SampleTime=6.25e-09  SaturateOnIntegerOverflow=off  InputSameDT=off
  adder : Sum  OutDataTypeStr=uint16  AccumDataTypeStr=uint16  SampleTime=6.25e-09
  compare : simulink/Logic and Bit Operations/Compare To Constant  relop===  const="fi(0,0,16,0,\"hex\",\"ffff\")"  OutDataTypeStr=boolean
  const : Constant  Value=0  VectorParams1D=off  OutDataTypeStr=uint16  SampleTime=6.25e-09
  countFrom : Constant  Value=0  VectorParams1D=off  OutDataTypeStr=uint16  SampleTime=6.25e-09
  crp_out_delay{,1..4} (5 alike) : Delay  DelayLength=double(1)  InitialCondition=0  SampleTime=6.25e-09
  "dataSelector " : Subsystem
  dataSelector 1 : RateTransition  InitialCondition=double(0)  OutPortSampleTimeOpt=Multiple of input port sample time  OutPortSampleTimeMultiple=8
  dataSelector 2 : RateTransition  InitialCondition=double(0)  OutPortSampleTimeOpt=Multiple of input port sample time  OutPortSampleTimeMultiple=8
  dataSelector 3 : RateTransition  InitialCondition=double(0)  OutPortSampleTimeOpt=Multiple of input port sample time  OutPortSampleTimeMultiple=8
  in0_repeat : RateTransition  Integrity=off  Deterministic=off  OutPortSampleTimeOpt=Multiple of input port sample time  OutPortSampleTimeMultiple=1/8
  in0_repeat1 : RateTransition  Integrity=off  Deterministic=off  OutPortSampleTimeOpt=Multiple of input port sample time  OutPortSampleTimeMultiple=1/8
  in1_repeat : RateTransition  Integrity=off  Deterministic=off  OutPortSampleTimeOpt=Multiple of input port sample time  OutPortSampleTimeMultiple=1/8
  in1_repeat1 : RateTransition  Integrity=off  Deterministic=off  OutPortSampleTimeOpt=Multiple of input port sample time  OutPortSampleTimeMultiple=1/8
  in2_repeat : RateTransition  Integrity=off  Deterministic=off  OutPortSampleTimeOpt=Multiple of input port sample time  OutPortSampleTimeMultiple=1/8
  in2_repeat1 : RateTransition  Integrity=off  Deterministic=off  OutPortSampleTimeOpt=Multiple of input port sample time  OutPortSampleTimeMultiple=1/8
  in3_repeat : RateTransition  Integrity=off  Deterministic=off  OutPortSampleTimeOpt=Multiple of input port sample time  OutPortSampleTimeMultiple=1/8
  in3_repeat1 : RateTransition  Integrity=off  Deterministic=off  OutPortSampleTimeOpt=Multiple of input port sample time  OutPortSampleTimeMultiple=1/8
  in4_repeat : RateTransition  Integrity=off  Deterministic=off  OutPortSampleTimeOpt=Multiple of input port sample time  OutPortSampleTimeMultiple=1/8
  in4_repeat1 : RateTransition  Integrity=off  Deterministic=off  OutPortSampleTimeOpt=Multiple of input port sample time  OutPortSampleTimeMultiple=1/8
  in5_repeat : RateTransition  Integrity=off  Deterministic=off  OutPortSampleTimeOpt=Multiple of input port sample time  OutPortSampleTimeMultiple=1/8
  in6_repeat : RateTransition  Integrity=off  Deterministic=off  OutPortSampleTimeOpt=Multiple of input port sample time  OutPortSampleTimeMultiple=1/8
  in7_repeat : RateTransition  Integrity=off  Deterministic=off  OutPortSampleTimeOpt=Multiple of input port sample time  OutPortSampleTimeMultiple=1/8
  rd_{1..3,7..10,31,51} (9 alike) : Delay  DelayLength=double(1)  InitialCondition=0  SampleTime=6.25e-09
  rd_4 : Delay  DelayLength=double(4)  InitialCondition=0  SampleTime=6.25e-09
  rd_5 : Delay  DelayLength=double(3)  InitialCondition=0  SampleTime=6.25e-09
  rd_6 : Delay  DelayLength=double(2)  InitialCondition=0  SampleTime=6.25e-09
  step_value : Constant  VectorParams1D=off  OutDataTypeStr=uint16  SampleTime=6.25e-09
  switch : Switch  Criteria=u2 ~= 0  Threshold="fi(0,0,1,0,\"hex\",\"0\")"  OutDataTypeStr=uint16  SampleTime=6.25e-09  SaturateOnIntegerOverflow=off  InputSameDT=off
  switchEnable : MultiPortSwitch  DataPortOrder=Zero-based contiguous  Inputs=2  DiagnosticForDefault=None  zeroidx=on  OutDataTypeStr=uint16  SampleTime=6.25e-09  SaturateOnIntegerOverflow=off  InputSameDT=off
  switchReset : Switch  Criteria=u2 ~= 0  Threshold="fi(0,0,1,0,\"hex\",\"0\")"  OutDataTypeStr=uint16  SampleTime=6.25e-09  SaturateOnIntegerOverflow=off  InputSameDT=off
  lstfStart : Outport  SampleTime=6.25e-09
  validOut : Outport  Port=2  SampleTime=6.25e-09
  dataOut : Outport  Port=3  SampleTime=5e-08
  wires:
  rd_1/1 -> Switch/1
  in2_repeat1/1 -> rd_1/1
  Delay11/1 -> Delay11_absorbed/1
  Logical Operator7/1 -> crp_out_delay3/1
  rd_2/1 -> Logical Operator7/1, Switch/2
  Delay12_absorbed/1 -> in4_repeat1/1
  Delay18/1 -> in6_repeat/1
  compare/1 -> rd_7/1
  in5_repeat/1 -> Relational Operator/1
  Logical Operator2/1 -> crp_out_delay2/1, Logical Operator3/1
  Delay11_absorbed/1 -> in2_repeat1/1
  dataIn/1 -> in1_repeat1/1
  counterRst/1 -> in3_repeat/1
  Logical Operator3/1 -> dataSelector 3/1, validOut/1
  Relational Operator/1 -> Logical Operator4/1
  in3_repeat1/1 -> rd_2/1
  in1_repeat1/1 -> Delay201/1
  dataSelector 3/1 -> "dataSelector "/1(syncEn)
  rd_5/1 -> switchEnable/1
  validIn/1 -> in2_repeat/1
  rd_51/1 -> Logical Operator6/2
  Delay20/1 -> in0_repeat/1
  in3_repeat/1 -> rd_4/1
  const/1 -> switchReset/1
  Switch/1 -> lstfStart/1
  switchReset/1 -> crp_out_delay1/1
  adder/1 -> rd_8/1
  HDL Counter2_absorbed/1 -> in4_repeat/1, Delay18/1
  in6_repeat/1 -> Relational Operator/2
  rd_3/1 -> compare/1, adder/1, rd_6/1
  HDL Counter2/1 -> HDL Counter2_absorbed/1
  crp_out_delay1/1 -> HDL Counter2/1
  step_value/1 -> adder/2
  maxPeakVal/1 -> in0_repeat1/1
  Delay17/1 -> Delay17_absorbed/1
  in4_repeat/1 -> rd_3/1
  rd_4/1 -> switchReset/2
  Delay21/1 -> in1_repeat/1
  in0_repeat1/1 -> crp_out_delay/1
  crp_out_delay/1 -> Delay17/1
  in1_repeat/1 -> Logical Operator4/2, dataSelector 2/1, Logical Operator3/2
  rd_8/1 -> switch/3
  in4_repeat1/1 -> rd_51/1
  in7_repeat/1 -> Logical Operator2/2
  in2_repeat/1 -> Delay211/1, rd_5/1
  Delay201/1 -> Delay20/1
  Logical Operator4/1 -> rd_31/1, Logical Operator2/1
  switch/1 -> rd_9/1
  rd_6/1 -> switchEnable/2
  dataSelector 2/1 -> "dataSelector "/3(validIn)
  rd_31/1 -> Logical Operator6/1, Switch/3, Logical Operator7/2
  rd_9/1 -> switchEnable/3
  crp_out_delay2/1 -> Delay7/1
  crp_out_delay3/1 -> Delay11/1
  Logical Operator6/1 -> crp_out_delay4/1
  in0_repeat/1 -> dataSelector 1/1
  Delay211/1 -> Delay21/1
  countFrom/1 -> switch/1
  switchEnable/1 -> rd_10/1
  Delay17_absorbed/1 -> in5_repeat/1
  dataSelector 1/1 -> "dataSelector "/2(dataIn)
  "dataSelector "/1(dataOut) -> dataOut/1
  crp_out_delay4/1 -> Delay10/1, Delay12/1
  rd_10/1 -> switchReset/3
  rd_7/1 -> switch/2
  Delay7/1 -> Delay7_absorbed/1
  Delay10/1 -> Delay10_absorbed/1
  Delay7_absorbed/1 -> in7_repeat/1
  Delay12/1 -> Delay12_absorbed/1
  Delay10_absorbed/1 -> in3_repeat1/1

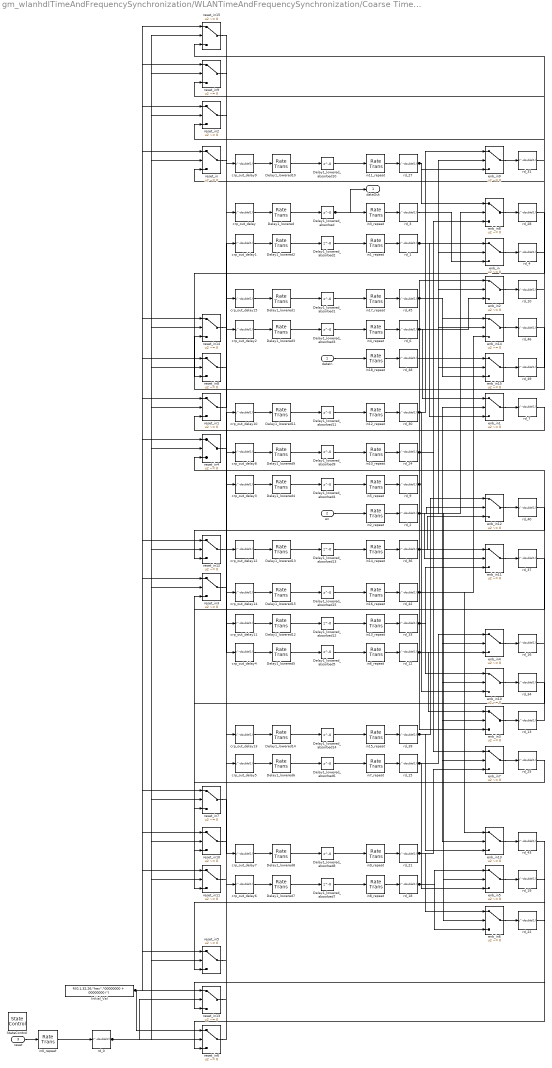
== system gm_wlanhdlTimeAndFrequencySynchronization/WLANTimeAndFrequencySynchronization/Coarse Time Sync/Correlator/MovingSum/Synchronous Enabled 128 Sample Delay  ==
  dataIn : Inport  OutDataTypeStr=fixdt(1, 32, 26)  PortDimensions=1  SampleTime=5e-08
      settings: SignalType=complex
  en : Inport  Port=2  OutDataTypeStr=boolean  PortDimensions=1  SampleTime=5e-08
  reset : Inport  Port=3  OutDataTypeStr=boolean  PortDimensions=1  SampleTime=5e-08
  Delay1_lowered{,1..15} (16 alike) : RateTransition  InitialCondition=double(0)  OutPortSampleTimeOpt=Multiple of input port sample time  OutPortSampleTimeMultiple=8
  Delay1_lowered_absorbed{,1..15} (16 alike) : Delay  DelayLength=0
  Initial_Val : Constant  Value="fi(0,1,32,26,\"hex\",\"00000000 + 00000000 i\")"  OutDataTypeStr=fixdt(1, 32, 26)  SampleTime=6.25e-09
  StateControl : StateControl  StateControl=Synchronous
  crp_out_delay{,1..15} (16 alike) : Delay  DelayLength=double(1)  InitialCondition=0  SampleTime=6.25e-09
  enb_in{,1..15} (16 alike) : Switch  Criteria=u2 ~= 0  Threshold=double(0)  OutDataTypeStr=fixdt(1, 32, 26)  SampleTime=6.25e-09  SaturateOnIntegerOverflow=off  InputSameDT=off
  in0_repeat : RateTransition  Integrity=off  Deterministic=off  OutPortSampleTimeOpt=Multiple of input port sample time  OutPortSampleTimeMultiple=1/8
  in10_repeat : RateTransition  Integrity=off  Deterministic=off  OutPortSampleTimeOpt=Multiple of input port sample time  OutPortSampleTimeMultiple=1/8
  in11_repeat : RateTransition  Integrity=off  Deterministic=off  OutPortSampleTimeOpt=Multiple of input port sample time  OutPortSampleTimeMultiple=1/8
  in12_repeat : RateTransition  Integrity=off  Deterministic=off  OutPortSampleTimeOpt=Multiple of input port sample time  OutPortSampleTimeMultiple=1/8
  in13_repeat : RateTransition  Integrity=off  Deterministic=off  OutPortSampleTimeOpt=Multiple of input port sample time  OutPortSampleTimeMultiple=1/8
  in14_repeat : RateTransition  Integrity=off  Deterministic=off  OutPortSampleTimeOpt=Multiple of input port sample time  OutPortSampleTimeMultiple=1/8
  in15_repeat : RateTransition  Integrity=off  Deterministic=off  OutPortSampleTimeOpt=Multiple of input port sample time  OutPortSampleTimeMultiple=1/8
  in16_repeat : RateTransition  Integrity=off  Deterministic=off  OutPortSampleTimeOpt=Multiple of input port sample time  OutPortSampleTimeMultiple=1/8
  in17_repeat : RateTransition  Integrity=off  Deterministic=off  OutPortSampleTimeOpt=Multiple of input port sample time  OutPortSampleTimeMultiple=1/8
  in18_repeat : RateTransition  Integrity=off  Deterministic=off  OutPortSampleTimeOpt=Multiple of input port sample time  OutPortSampleTimeMultiple=1/8
  in1_repeat : RateTransition  Integrity=off  Deterministic=off  OutPortSampleTimeOpt=Multiple of input port sample time  OutPortSampleTimeMultiple=1/8
  in2_repeat : RateTransition  Integrity=off  Deterministic=off  OutPortSampleTimeOpt=Multiple of input port sample time  OutPortSampleTimeMultiple=1/8
  in3_repeat : RateTransition  Integrity=off  Deterministic=off  OutPortSampleTimeOpt=Multiple of input port sample time  OutPortSampleTimeMultiple=1/8
  in4_repeat : RateTransition  Integrity=off  Deterministic=off  OutPortSampleTimeOpt=Multiple of input port sample time  OutPortSampleTimeMultiple=1/8
  in5_repeat : RateTransition  Integrity=off  Deterministic=off  OutPortSampleTimeOpt=Multiple of input port sample time  OutPortSampleTimeMultiple=1/8
  in6_repeat : RateTransition  Integrity=off  Deterministic=off  OutPortSampleTimeOpt=Multiple of input port sample time  OutPortSampleTimeMultiple=1/8
  in7_repeat : RateTransition  Integrity=off  Deterministic=off  OutPortSampleTimeOpt=Multiple of input port sample time  OutPortSampleTimeMultiple=1/8
  in8_repeat : RateTransition  Integrity=off  Deterministic=off  OutPortSampleTimeOpt=Multiple of input port sample time  OutPortSampleTimeMultiple=1/8
  in9_repeat : RateTransition  Integrity=off  Deterministic=off  OutPortSampleTimeOpt=Multiple of input port sample time  OutPortSampleTimeMultiple=1/8
  rd_0 : Delay  DelayLength=double(2)  InitialCondition=0  SampleTime=6.25e-09
  rd_{1..4,6..7,9..10,12..13,15..16,18..19,21..22,24..25,27..28,30..31,33..34,36..37,39..40,42..43,45..46,48..49} (34 alike) : Delay  DelayLength=double(1)  InitialCondition=0  SampleTime=6.25e-09
  reset_in{,1..15} (16 alike) : Switch  Criteria=u2 ~= 0  Threshold=double(0)  OutDataTypeStr=fixdt(1, 32, 26)  SampleTime=6.25e-09  SaturateOnIntegerOverflow=off  InputSameDT=off
  dataOut : Outport  SampleTime=5e-08  VectorParamsAs1DForOutWhenUnconnected=off
  wires:
  rd_48/1 -> enb_in15/1
  crp_out_delay9/1 -> Delay1_lowered10/1
  crp_out_delay8/1 -> Delay1_lowered9/1
  Delay1_lowered_absorbed2/1 -> in1_repeat/1
  rd_42/1 -> enb_in13/1, enb_in14/3
  Delay1_lowered1/1 -> Delay1_lowered_absorbed1/1
  enb_in8/1 -> rd_28/1
  Delay1_lowered_absorbed11/1 -> in12_repeat/1
  crp_out_delay11/1 -> Delay1_lowered12/1
  Delay1_lowered12/1 -> Delay1_lowered_absorbed12/1
  crp_out_delay7/1 -> Delay1_lowered8/1
  Delay1_lowered_absorbed/1 -> in3_repeat/1, dataOut/1
  crp_out_delay5/1 -> Delay1_lowered6/1
  enb_in12/1 -> rd_40/1
  reset_in3/1 -> crp_out_delay3/1
  Delay1_lowered_absorbed14/1 -> in15_repeat/1
  rd_15/1 -> enb_in5/3, enb_in4/1
  Initial_Val/1 -> reset_in1/1, reset_in2/1, reset_in3/1, reset_in4/1, reset_in5/1, reset_in11/1, reset_in12/1, reset_in6/1, reset_in9/1, reset_in7/1, reset_in8/1, reset_in10/1, reset_in15/1, reset_in14/1, reset_in13/1, reset_in/1
  Delay1_lowered8/1 -> Delay1_lowered_absorbed8/1
  in18_repeat/1 -> rd_48/1
  Delay1_lowered_absorbed1/1 -> in17_repeat/1
  rd_49/1 -> reset_in15/3
  Delay1_lowered10/1 -> Delay1_lowered_absorbed10/1
  enb_in10/1 -> rd_34/1
  Delay1_lowered3/1 -> Delay1_lowered_absorbed3/1
  in6_repeat/1 -> rd_12/1
  reset_in13/1 -> crp_out_delay13/1
  enb_in13/1 -> rd_43/1
  Delay1_lowered_absorbed9/1 -> in10_repeat/1
  rd_2/1 -> enb_in11/2, enb_in15/2, enb_in14/2, enb_in9/2, enb_in7/2, enb_in6/2, enb_in5/2, enb_in4/2, enb_in3/2, enb_in/2, enb_in2/2, enb_in13/2, enb_in1/2, enb_in8/2, enb_in12/2, enb_in10/2
  in0_repeat/1 -> rd_0/1
  Delay1_lowered2/1 -> Delay1_lowered_absorbed2/1
  rd_13/1 -> reset_in3/3
  crp_out_delay14/1 -> Delay1_lowered15/1
  Delay1_lowered_absorbed6/1 -> in7_repeat/1
  rd_16/1 -> reset_in4/3
  Delay1_lowered_absorbed13/1 -> in14_repeat/1
  rd_34/1 -> reset_in10/3
  rd_25/1 -> reset_in7/3
  crp_out_delay2/1 -> Delay1_lowered3/1
  rd_19/1 -> reset_in5/3
  rd_12/1 -> enb_in3/1, enb_in4/3
  crp_out_delay/1 -> Delay1_lowered/1
  rd_10/1 -> reset_in2/3
  rd_22/1 -> reset_in6/3
  enb_in15/1 -> rd_49/1
  rd_37/1 -> reset_in11/3
  rd_40/1 -> reset_in12/3
  rd_39/1 -> enb_in12/1, enb_in13/3
  reset_in11/1 -> crp_out_delay11/1
  crp_out_delay10/1 -> Delay1_lowered11/1
  enb_in5/1 -> rd_19/1
  rd_28/1 -> reset_in8/3
  rd_3/1 -> enb_in/3
  enb_in14/1 -> rd_46/1
  Delay1_lowered_absorbed8/1 -> in9_repeat/1
  Delay1_lowered_absorbed5/1 -> in6_repeat/1
  en/1 -> in2_repeat/1
  enb_in7/1 -> rd_25/1
  enb_in11/1 -> rd_37/1
  reset_in10/1 -> crp_out_delay10/1
  enb_in4/1 -> rd_16/1
  Delay1_lowered7/1 -> Delay1_lowered_absorbed7/1
  reset_in1/1 -> crp_out_delay1/1
  Delay1_lowered13/1 -> Delay1_lowered_absorbed13/1
  rd_21/1 -> enb_in6/1, enb_in7/3
  in16_repeat/1 -> rd_42/1
  rd_7/1 -> reset_in1/3
  in15_repeat/1 -> rd_39/1
  enb_in2/1 -> rd_10/1
  in3_repeat/1 -> rd_3/1
  rd_46/1 -> reset_in14/3
  rd_0/1 -> reset_in11/2, reset_in10/2, reset_in15/2, reset_in13/2, reset_in12/2, reset_in14/2, reset_in7/2, reset_in5/2, reset_in2/2, reset_in/2, reset_in9/2, reset_in8/2, reset_in6/2, reset_in1/2, reset_in3/2, reset_in4/2
  reset_in7/1 -> crp_out_delay7/1
  in1_repeat/1 -> rd_1/1
  Delay1_lowered6/1 -> Delay1_lowered_absorbed6/1
  Delay1_lowered_absorbed4/1 -> in5_repeat/1
  in10_repeat/1 -> rd_24/1
  rd_45/1 -> enb_in15/3, enb_in14/1
  in12_repeat/1 -> rd_30/1
  reset_in15/1 -> crp_out_delay15/1
  reset_in/1 -> crp_out_delay/1
  rd_31/1 -> reset_in9/3
  rd_6/1 -> enb_in2/3, enb_in1/1
  dataIn/1 -> in18_repeat/1
  rd_36/1 -> enb_in11/1, enb_in12/3
  crp_out_delay15/1 -> Delay1_lowered1/1
  in9_repeat/1 -> rd_21/1
  Delay1_lowered5/1 -> Delay1_lowered_absorbed5/1
  Delay1_lowered14/1 -> Delay1_lowered_absorbed14/1
  reset_in12/1 -> crp_out_delay12/1
  rd_4/1 -> reset_in/3
  rd_27/1 -> enb_in9/3, enb_in8/1
  in5_repeat/1 -> rd_9/1
  rd_1/1 -> enb_in1/3, enb_in/1
  reset_in4/1 -> crp_out_delay4/1
  in4_repeat/1 -> rd_6/1
  crp_out_delay3/1 -> Delay1_lowered4/1
  Delay1_lowered_absorbed15/1 -> in16_repeat/1
  Delay1_lowered4/1 -> Delay1_lowered_absorbed4/1
  in11_repeat/1 -> rd_27/1
  rd_9/1 -> enb_in2/1, enb_in3/3
  crp_out_delay13/1 -> Delay1_lowered14/1
  crp_out_delay1/1 -> Delay1_lowered2/1
  reset/1 -> in0_repeat/1
  reset_in14/1 -> crp_out_delay14/1
  in2_repeat/1 -> rd_2/1
  crp_out_delay12/1 -> Delay1_lowered13/1
  enb_in3/1 -> rd_13/1
  enb_in6/1 -> rd_22/1
  enb_in/1 -> rd_4/1
  Delay1_lowered_absorbed12/1 -> in13_repeat/1
  Delay1_lowered9/1 -> Delay1_lowered_absorbed9/1
  Delay1_lowered15/1 -> Delay1_lowered_absorbed15/1
  Delay1_lowered/1 -> Delay1_lowered_absorbed/1
  Delay1_lowered_absorbed3/1 -> in4_repeat/1
  Delay1_lowered_absorbed10/1 -> in11_repeat/1
  rd_30/1 -> enb_in9/1, enb_in10/3
  enb_in9/1 -> rd_31/1
  reset_in9/1 -> crp_out_delay9/1
  rd_43/1 -> reset_in13/3
  in8_repeat/1 -> rd_18/1
  Delay1_lowered_absorbed7/1 -> in8_repeat/1
  reset_in2/1 -> crp_out_delay2/1
  crp_out_delay4/1 -> Delay1_lowered5/1
  in7_repeat/1 -> rd_15/1
  enb_in1/1 -> rd_7/1
  reset_in5/1 -> crp_out_delay5/1
  reset_in6/1 -> crp_out_delay6/1
  rd_33/1 -> enb_in10/1, enb_in11/3
  crp_out_delay6/1 -> Delay1_lowered7/1
  reset_in8/1 -> crp_out_delay8/1
  Delay1_lowered11/1 -> Delay1_lowered_absorbed11/1
  in17_repeat/1 -> rd_45/1
  in13_repeat/1 -> rd_33/1
  rd_24/1 -> enb_in8/3, enb_in7/1
  in14_repeat/1 -> rd_36/1
  rd_18/1 -> enb_in6/3, enb_in5/1

== system gm_wlanhdlTimeAndFrequencySynchronization/WLANTimeAndFrequencySynchronization/Coarse Time Sync/Correlator/delayedCorrelation/DTadjust ==
  in : Inport  OutDataTypeStr=fixdt(1, 32, 24)  PortDimensions=1  SampleTime=5e-08
      settings: SignalType=complex
  DTadjust : MATLAB Function  TreatAsAtomicUnit=on
  out : Outport  SampleTime=5e-08  VectorParamsAs1DForOutWhenUnconnected=off
  wires:
  DTadjust/1(out) -> out/1
  in/1 -> DTadjust/1(in)
